simulink model "labels"  (R2014a)
settings: Solver=ode45  StartTime=0.0  StopTime=10.0  RelTol=1e-3
settings Model: Creator=ladmin  LastModifiedBy=ladmin

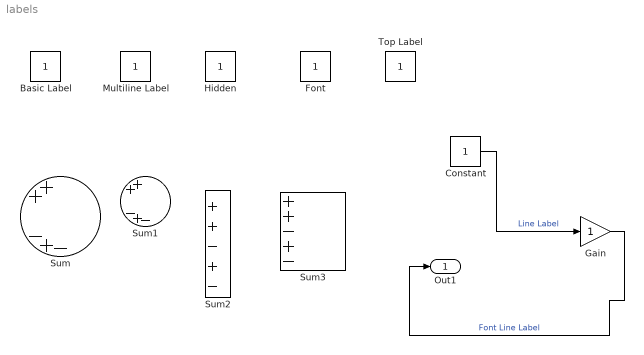
== system labels ==
  Basic Label : Constant
  Constant : Constant
  Font : Constant
  Gain : Gain
  Hidden : Constant
  Multiline Label : Constant
  Sum{,1..3} (4 alike) : Sum  Inputs=|++||-+-
  Top Label : Constant
  Out1 : Outport
  wires:
  Constant/1 -> Gain/1  "Line Label"
  Gain/1 -> Out1/1  "Font Line Label"
